simulink model "Simulink_example_01"  (R2023a)
settings: Solver=VariableStepAuto  StartTime=0.0  StopTime=10.0  RelTol=1e-3
libraries: simulink x1
settings Model: Creator=hsllo  LastModifiedBy=hsllo

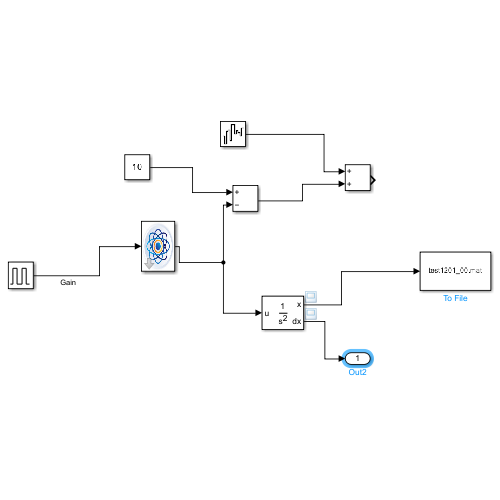
[thumbnail: Simulink's stored preview of the top-level diagram]
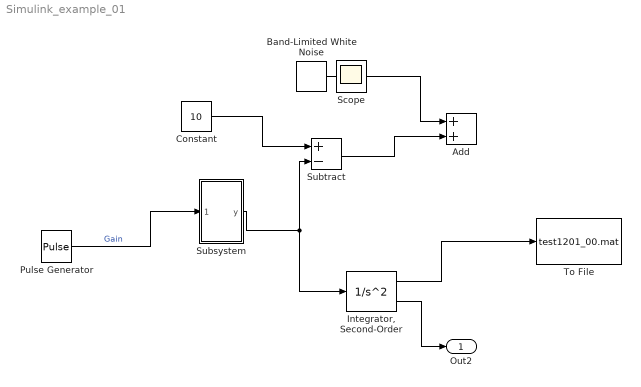
== system Simulink_example_01 ==
  Add : Sum
  Band-Limited White Noise : simulink/Sources/Band-Limited White Noise  Cov=[0.1]  Ts=0.1  seed=[23341]
  Constant : Constant  Value=10
  "Integrator, Second-Order" : SecondOrderIntegrator
  Pulse Generator : DiscretePulseGenerator  PulseType=Time based  Period=10  PulseWidth=5
  Subsystem : Subsystem
      mask DialogControl ParameterGroupVar Prompt: 파라미터
      mask Display: image('mask01.jpg');
  Subtract : Sum  Inputs=+-
  To File : ToFile  Filename=test1201_00.mat  SaveFormat=Timeseries
  Out2 : Outport
  Scope : Scope
  wires:
  Pulse Generator/1 -> Subsystem/1(Gain1)  "Gain"
  Subsystem/1(y) -> "Integrator, Second-Order"/1, Subtract/2
  "Integrator, Second-Order"/1 -> To File/1
  "Integrator, Second-Order"/2 -> Out2/1
  Constant/1 -> Subtract/1
  Subtract/1 -> Add/2
  Band-Limited White Noise/1 -> Add/1

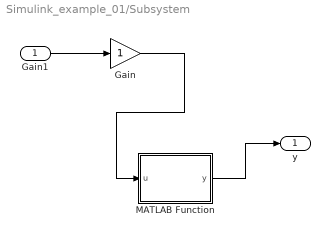
== system Simulink_example_01/Subsystem ==
  Gain1 : Inport
  Gain : Gain
  MATLAB Function : MATLAB Function  TreatAsAtomicUnit=on
  y : Outport
  wires:
  Gain/1 -> MATLAB Function/1(u)
  Gain1/1 -> Gain/1
  MATLAB Function/1(y) -> y/1

== matlab function Simulink_example_01/Subsystem/MATLAB Function ==
  data: u input; y output
function y = fcn(u)

y = u*rand();
